simulink model "Model_V9"  (R2024a)
settings: Solver=FixedStepAuto  StartTime=0.0  StopTime=15  FixedStep=10^-3  RelTol=1e-3
values from neighbouring files (symbols this model uses):
  a1 = 1.6552    [varglobal.m]
  a2 = 1.885    [varglobal.m]
  b1 = 0.71    [varglobal.m]
  b2 = 0.71    [varglobal.m]
  Ga1 = 1/7    (= 0.142857142857)    [varglobal.m]
  Gu1 = 1.8    [varglobal.m]
  Gv1 = 1/0.5    (= 2)    [varglobal.m]
  Gx1 = 1/0.5    (= 2)    [varglobal.m]
undefined symbols (not defined in the file or in its folder): eqmovimento, Forcalateral, ForcaMolaFrontal, ForcaMolaRetaguarda, Rotacao, Saidas, sigbuilder_block, Transformador, TransformadorT
libraries: simulink_extras x5, fuzblock x4
settings Model: Creator=Vilson Wenis Belle  LastModifiedBy=wenis
settings SolverCC: AlgebraicLoopSolver=TrustRegion
settings DebuggingCC: UnconnectedInputMsg=warning  UnconnectedOutputMsg=warning  UnconnectedLineMsg=warning
settings ModelReferenceCC: EnableRefExpFcnMdlSchedulingChecks=on
settings RTWCC: GPUComputeCapability=3.5

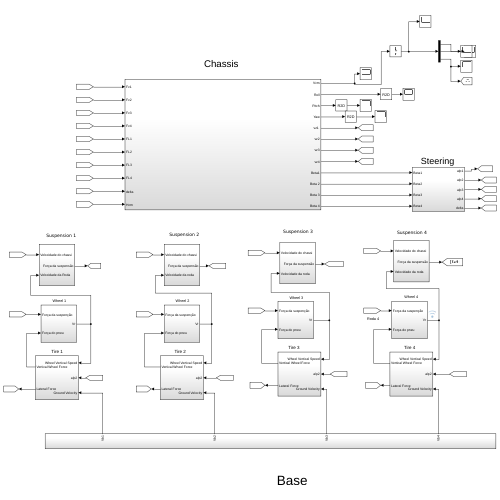
[thumbnail: Simulink's stored preview of the top-level diagram]
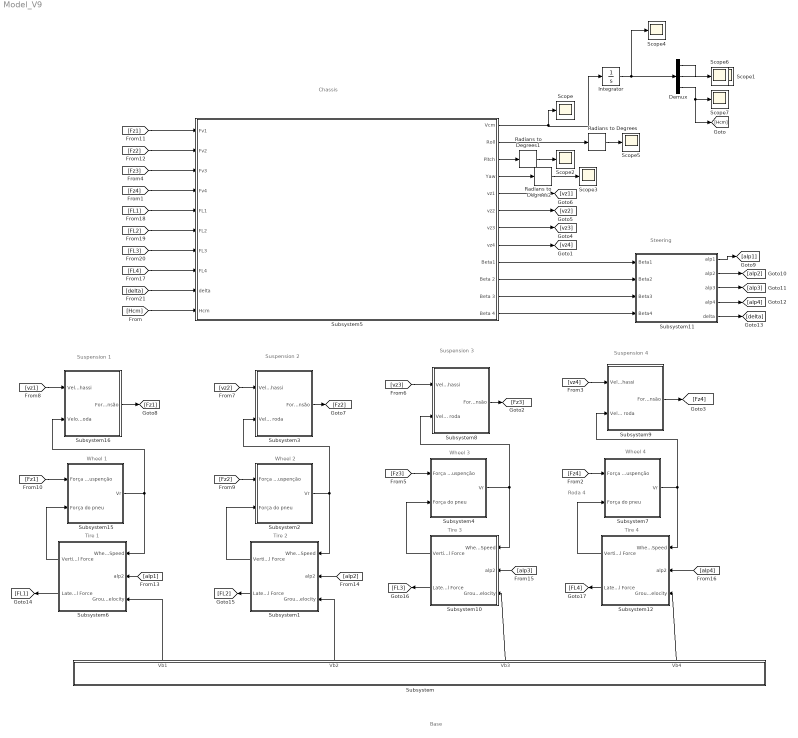
== system Model_V9 ==
  note: Chassis
  note: Steering
  note: Suspension 4
  note: Roda 4
  note: Tire 4
  note: Suspension 3
  note: Wheel 3
  note: Suspension 2
  note: Wheel 2
  note: Base
  note: Suspension 1
  note: Wheel 1
  note: Tire 3
  note: Tire 2
  note: Tire 1
  note: Wheel 4
  Demux : Demux  Outputs=3
  Integrator : Integrator  InitialCondition=[0 (1.1*1.4 + 0.25)/2 0.6]
  Radians to Degrees : simulink_extras/Transformations/Radians to Degrees
  Radians to Degrees1 : simulink_extras/Transformations/Radians to Degrees
  Radians to Degrees2 : simulink_extras/Transformations/Radians to Degrees
  Scope{,1..7} (8 alike) : Scope
  Subsystem : Subsystem
  Subsystem1 : Subsystem
  Subsystem10 : Subsystem
  Subsystem11 : Subsystem
  Subsystem12 : Subsystem
  Subsystem15 : Subsystem
  Subsystem16 : Subsystem
  Subsystem2 : Subsystem
  Subsystem3 : Subsystem
  Subsystem4 : Subsystem
  Subsystem5 : Subsystem
  Subsystem6 : Subsystem
  Subsystem7 : Subsystem
  Subsystem8 : Subsystem
  Subsystem9 : Subsystem
  wires:
  Subsystem12/1(Vertical Wheel Force) -> Subsystem7/2(Força do pneu)
  Subsystem7/1(Vr) -> Subsystem12/1(Wheel Vertical Speed), Subsystem9/2(Velocidade da roda)
  Subsystem4/1(Vr) -> Subsystem10/1(Wheel Vertical Speed), Subsystem8/2(Velocidade da roda)
  Subsystem10/1(Vertical Wheel Force) -> Subsystem4/2(Força do pneu)
  Subsystem2/1(Vr) -> Subsystem1/1(Wheel Vertical Speed), Subsystem3/2(Velocidade da roda)
  Subsystem1/1(Vertical Wheel Force) -> Subsystem2/2(Força do pneu)
  Subsystem15/1(Vr) -> Subsystem6/1(Wheel Vertical Speed), Subsystem16/2(Velocidade da Roda)
  Subsystem9/1(Força da suspensão) -> [Fz4]
  Subsystem5/1(Vcm) -> Scope/1, Integrator/1
  Subsystem5/2(Roll) -> Radians to Degrees/1
  Subsystem5/3(Pitch) -> Radians to Degrees1/1
  Subsystem5/4(Yaw) -> Radians to Degrees2/1
  Integrator/1 -> Scope4/1, Demux/1
  Subsystem6/1(Vertical Wheel Force) -> Subsystem15/2(Força do pneu)
  [Fz4] -> Subsystem5/4(Fv4)
  [Fz4] -> Subsystem7/1(Força da suspenção)
  Subsystem5/8(vz4) -> [vz4]
  [vz4] -> Subsystem9/1(Velocidade do chassi)
  [Fz3] -> Subsystem5/3(Fv3)
  Subsystem8/1(Força da suspensão) -> [Fz3]
  [Fz3] -> Subsystem4/1(Força da suspenção)
  Subsystem5/7(vz3) -> [vz3]
  [vz3] -> Subsystem8/1(Velocidade do chassi)
  Subsystem5/6(vz2) -> [vz2]
  Subsystem5/5("vz1 ") -> [vz1]
  [vz2] -> Subsystem3/1(Velocidade do chassi)
  [vz1] -> Subsystem16/1(Velocidade do chassi)
  Subsystem3/1(Força da suspensão) -> [Fz2]
  Subsystem16/1(Força da suspensão) -> [Fz1]
  [Fz2] -> Subsystem2/1(Força da suspenção)
  [Fz1] -> Subsystem15/1(Força da suspenção)
  [Fz1] -> Subsystem5/1(Fv1)
  [Fz2] -> Subsystem5/2(Fv2)
  Subsystem/1(Vb1) -> Subsystem6/3(Ground Velocity)
  Subsystem/2(Vb2) -> Subsystem1/3(Ground Velocity)
  Subsystem/3(Vb3) -> Subsystem10/3(Ground Velocity)
  Subsystem/4(Vb4) -> Subsystem12/3(Ground Velocity)
  Subsystem5/9(Beta1) -> Subsystem11/1("Beta1 ")
  Subsystem5/10(Beta 2) -> Subsystem11/2(Beta2)
  Subsystem5/11(Beta 3) -> Subsystem11/3(Beta3)
  Subsystem5/12(Beta 4) -> Subsystem11/4(Beta4)
  [alp1] -> Subsystem6/2(alp2)
  Subsystem11/1(alp1) -> [alp1]
  Subsystem11/2(alp2) -> [alp2]
  Subsystem11/3(alp3) -> [alp3]
  Subsystem11/4(alp4) -> [alp4]
  Subsystem11/5(delta) -> [delta]
  [alp2] -> Subsystem1/2(alp2)
  [alp3] -> Subsystem10/2(alp2)
  [alp4] -> Subsystem12/2(alp2)
  Subsystem6/2(Lateral Force) -> [FL1]
  Subsystem1/2(Lateral Force) -> [FL2]
  Subsystem10/2(Lateral Force) -> [FL3]
  Subsystem12/2(Lateral Force) -> [FL4]
  [FL1] -> Subsystem5/5(FL1)
  [FL2] -> Subsystem5/6(FL2)
  [FL3] -> Subsystem5/7(FL3)
  [FL4] -> Subsystem5/8(FL4)
  [delta] -> Subsystem5/9(delta)
  Radians to Degrees1/1 -> Scope2/1
  Demux/1 -> Scope1/1
  Demux/2 -> Scope6/1
  Demux/3 -> [Hcm], Scope7/1
  [Hcm] -> Subsystem5/10("Hcm ")
  Radians to Degrees2/1 -> Scope3/1
  Radians to Degrees/1 -> Scope5/1

== system Model_V9/Subsystem ==
  Signal Builder : Subsystem  Tag=STV Subsys  LoadFcn=sigbuilder_block('load');  StartFcn=sigbuilder_block('start');  StopFcn=sigbuilder_block('stop');  ClipboardFcn=sigbuilder_block('clipboard');  mask(Sigbuilder block){tuvar=[0:10]}
      mask help: Simulink:masks:SigbuilderBlock_MD
      mask init:
      | if ~strcmp(get_param(bdroot(gcbh),'SimulationStatus'),'stopped') tuvar = sigbuilder_block('maskInit'); end
      settings: CopyFcn=sigbuilder_block('copy');  DeleteFcn=sigbuilder_block('delete');  ModelCloseFcn=sigbuilder_block('modelClose');  PreSaveFcn=sigbuilder_block('preSave');  PauseFcn=sigbuilder_block('pause');  ContinueFcn=sigbuilder_block('continue');  NameChangeFcn=sigbuilder_block('namechange');  OpenFcn=sigbuilder_block('open',[437.25 153 550.5 359.25 ]);  CloseFcn=sigbuilder_block('close');
      mask Display: plot(0, 0, 100, 100,[2, 2, 32, 32, 2], [68, 8, 8, 68, 68],[32, 2], [38, 38], [32, 19, 2],[53, 60, 44], [32, 17, 17, 2],[16, 16, 31, 31]);txt = getActiveGroup(gcbh);text(2, 100, txt,'verticalAlignment', 'top');
  Vb1 : Outport
  Vb2 : Outport  Port=2
  Vb3 : Outport  Port=3
  Vb4 : Outport  Port=4
  wires:
  Signal Builder/1(Signal 1) -> Vb1/1
  Signal Builder/2(Signal 2) -> Vb2/1
  Signal Builder/3(Signal 3) -> Vb3/1
  Signal Builder/4(Signal 4) -> Vb4/1

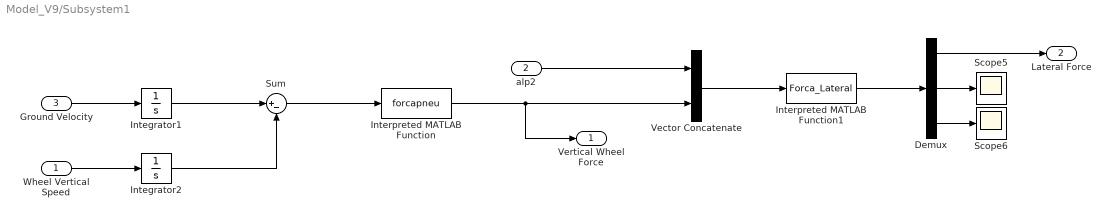
== system Model_V9/Subsystem1 ==
  Wheel Vertical Speed : Inport
  alp2 : Inport  Port=2
  Ground Velocity : Inport  Port=3
  Demux : Demux  Outputs=3
  Integrator1 : Integrator
  Integrator2 : Integrator
  Interpreted MATLAB Function : MATLABFcn  MATLABFcn=forcapneu  OutputDimensions=1
  Interpreted MATLAB Function1 : MATLABFcn  MATLABFcn=Forca_Lateral  OutputDimensions=3
  Scope5 : Scope
  Scope6 : Scope
  Sum : Sum  Inputs=|+-
  Vector Concatenate : Concatenate
  Vertical Wheel Force : Outport
  Lateral Force : Outport  Port=2
  wires:
  Ground Velocity/1 -> Integrator1/1
  Integrator2/1 -> Sum/2
  Interpreted MATLAB Function/1 -> Vertical Wheel Force/1, Vector Concatenate/2
  Integrator1/1 -> Sum/1
  Wheel Vertical Speed/1 -> Integrator2/1
  Sum/1 -> Interpreted MATLAB Function/1
  alp2/1 -> Vector Concatenate/1
  Vector Concatenate/1 -> Interpreted MATLAB Function1/1
  Interpreted MATLAB Function1/1 -> Demux/1
  Demux/1 -> Lateral Force/1
  Demux/2 -> Scope5/1
  Demux/3 -> Scope6/1

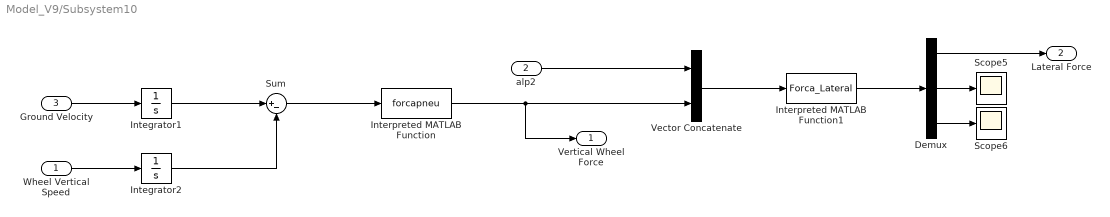
== system Model_V9/Subsystem10 ==
  Wheel Vertical Speed : Inport
  alp2 : Inport  Port=2
  Ground Velocity : Inport  Port=3
  Demux : Demux  Outputs=3
  Integrator1 : Integrator
  Integrator2 : Integrator
  Interpreted MATLAB Function : MATLABFcn  MATLABFcn=forcapneu  OutputDimensions=1
  Interpreted MATLAB Function1 : MATLABFcn  MATLABFcn=Forca_Lateral  OutputDimensions=3
  Scope5 : Scope
  Scope6 : Scope
  Sum : Sum  Inputs=|+-
  Vector Concatenate : Concatenate
  Vertical Wheel Force : Outport
  Lateral Force : Outport  Port=2
  wires:
  Ground Velocity/1 -> Integrator1/1
  Integrator2/1 -> Sum/2
  Interpreted MATLAB Function/1 -> Vertical Wheel Force/1, Vector Concatenate/2
  Integrator1/1 -> Sum/1
  Wheel Vertical Speed/1 -> Integrator2/1
  Sum/1 -> Interpreted MATLAB Function/1
  alp2/1 -> Vector Concatenate/1
  Vector Concatenate/1 -> Interpreted MATLAB Function1/1
  Interpreted MATLAB Function1/1 -> Demux/1
  Demux/1 -> Lateral Force/1
  Demux/2 -> Scope5/1
  Demux/3 -> Scope6/1

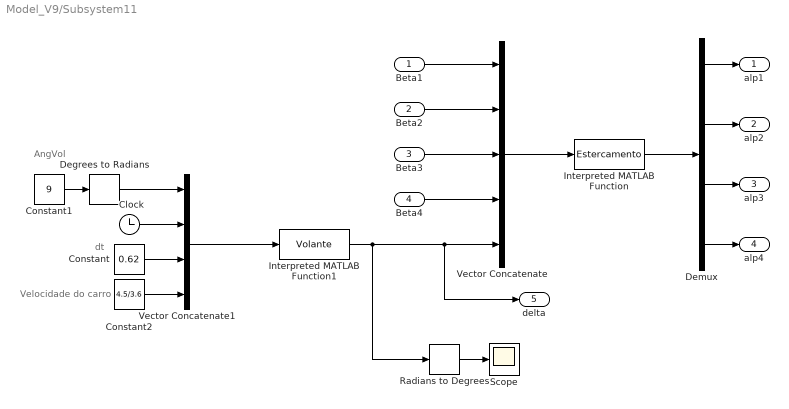
== system Model_V9/Subsystem11 ==
  note: Velocidade do carro
  note: dt
  note: AngVol
  "Beta1 " : Inport
  Beta2 : Inport  Port=2
  Beta3 : Inport  Port=3
  Beta4 : Inport  Port=4
  Clock : Clock
  Constant : Constant  Value=0.62
  Constant1 : Constant  Value=9
  Constant2 : Constant  Value=4.5/3.6
  Degrees to Radians : simulink_extras/Transformations/Degrees to Radians
  Demux : Demux
  Interpreted MATLAB Function : MATLABFcn  MATLABFcn=Estercamento  OutputDimensions=4
  Interpreted MATLAB Function1 : MATLABFcn  MATLABFcn=Volante  OutputDimensions=1
  Radians to Degrees : simulink_extras/Transformations/Radians to Degrees
  Scope : Scope
  Vector Concatenate : Concatenate  NumInputs=5
  Vector Concatenate1 : Concatenate  NumInputs=4
  alp1 : Outport
  alp2 : Outport  Port=2
  alp3 : Outport  Port=3
  alp4 : Outport  Port=4
  delta : Outport  Port=5
  wires:
  Beta4/1 -> Vector Concatenate/4
  Beta3/1 -> Vector Concatenate/3
  Beta2/1 -> Vector Concatenate/2
  "Beta1 "/1 -> Vector Concatenate/1
  Vector Concatenate/1 -> Interpreted MATLAB Function/1
  Interpreted MATLAB Function/1 -> Demux/1
  Demux/1 -> alp1/1
  Demux/2 -> alp2/1
  Demux/3 -> alp3/1
  Demux/4 -> alp4/1
  Clock/1 -> Vector Concatenate1/2
  Constant1/1 -> Degrees to Radians/1
  Constant/1 -> Vector Concatenate1/3
  Vector Concatenate1/1 -> Interpreted MATLAB Function1/1
  Degrees to Radians/1 -> Vector Concatenate1/1
  Constant2/1 -> Vector Concatenate1/4
  Radians to Degrees/1 -> Scope/1
  Interpreted MATLAB Function1/1 -> delta/1, Vector Concatenate/5, Radians to Degrees/1

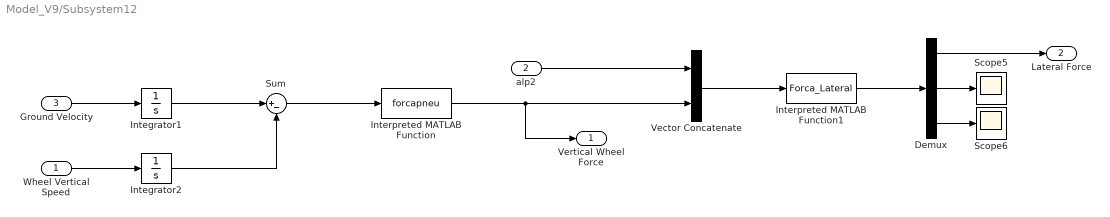
== system Model_V9/Subsystem12 ==
  Wheel Vertical Speed : Inport
  alp2 : Inport  Port=2
  Ground Velocity : Inport  Port=3
  Demux : Demux  Outputs=3
  Integrator1 : Integrator
  Integrator2 : Integrator
  Interpreted MATLAB Function : MATLABFcn  MATLABFcn=forcapneu  OutputDimensions=1
  Interpreted MATLAB Function1 : MATLABFcn  MATLABFcn=Forca_Lateral  OutputDimensions=3
  Scope5 : Scope
  Scope6 : Scope
  Sum : Sum  Inputs=|+-
  Vector Concatenate : Concatenate
  Vertical Wheel Force : Outport
  Lateral Force : Outport  Port=2
  wires:
  Ground Velocity/1 -> Integrator1/1
  Integrator2/1 -> Sum/2
  Interpreted MATLAB Function/1 -> Vertical Wheel Force/1, Vector Concatenate/2
  Integrator1/1 -> Sum/1
  Wheel Vertical Speed/1 -> Integrator2/1
  Sum/1 -> Interpreted MATLAB Function/1
  alp2/1 -> Vector Concatenate/1
  Vector Concatenate/1 -> Interpreted MATLAB Function1/1
  Interpreted MATLAB Function1/1 -> Demux/1
  Demux/1 -> Lateral Force/1
  Demux/2 -> Scope5/1
  Demux/3 -> Scope6/1

== system Model_V9/Subsystem15 ==
  Força da suspenção : Inport
  Força do pneu : Inport  Port=2
  Integrator : Integrator
  Interpreted MATLAB Function1 : MATLABFcn  MATLABFcn=aceleracaorodafrontal  OutputDimensions=1
  Sum : Sum  Inputs=|-+
  Vr : Outport
  wires:
  Força da suspenção/1 -> Sum/1
  Força do pneu/1 -> Sum/2
  Integrator/1 -> Vr/1
  Sum/1 -> Interpreted MATLAB Function1/1
  Interpreted MATLAB Function1/1 -> Integrator/1

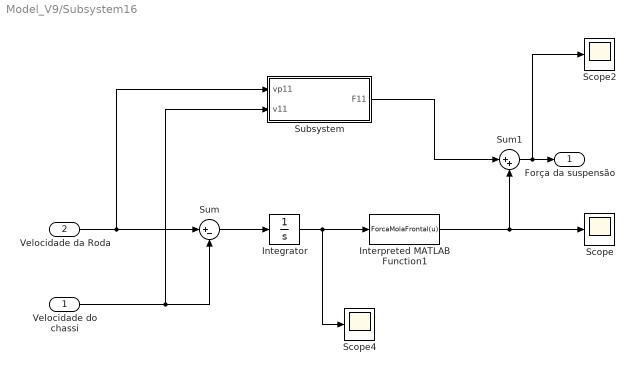
== system Model_V9/Subsystem16 ==
  Velocidade do chassi : Inport
  Velocidade da Roda : Inport  Port=2
  Integrator : Integrator
  Interpreted MATLAB Function1 : MATLABFcn  MATLABFcn=ForcaMolaFrontal(u)  OutputDimensions=1
  Scope : Scope
  Scope2 : Scope
  Scope4 : Scope
  Subsystem : Subsystem
  Sum : Sum  Inputs=|+-
  Sum1 : Sum  Inputs=|++
  Força da suspensão : Outport
  wires:
  Velocidade do chassi/1 -> Subsystem/2(v11), Sum/2
  Velocidade da Roda/1 -> Subsystem/1(vp11), Sum/1
  Sum/1 -> Integrator/1
  Integrator/1 -> Scope4/1, Interpreted MATLAB Function1/1
  Interpreted MATLAB Function1/1 -> Scope/1, Sum1/2
  Sum1/1 -> Scope2/1, Força da suspensão/1
  Subsystem/1(F11) -> Sum1/1

== system Model_V9/Subsystem2 ==
  Força da suspenção : Inport
  Força do pneu : Inport  Port=2
  Integrator : Integrator
  Interpreted MATLAB Function : MATLABFcn  MATLABFcn=aceleracaorodafrontal  OutputDimensions=1
  Sum : Sum  Inputs=|-+
  Vr : Outport
  wires:
  Força da suspenção/1 -> Sum/1
  Força do pneu/1 -> Sum/2
  Integrator/1 -> Vr/1
  Sum/1 -> Interpreted MATLAB Function/1
  Interpreted MATLAB Function/1 -> Integrator/1

== system Model_V9/Subsystem3 ==
  Velocidade do chassi : Inport
  Velocidade da roda : Inport  Port=2
  Integrator : Integrator
  Interpreted MATLAB Function1 : MATLABFcn  MATLABFcn=ForcaMolaFrontal(u)  OutputDimensions=1
  Scope : Scope
  Scope1 : Scope
  Scope2 : Scope
  Subsystem : Subsystem
  Sum : Sum  Inputs=|+-
  Sum1 : Sum  Inputs=|++
  Força da suspensão : Outport
  wires:
  Velocidade do chassi/1 -> Subsystem/2(v11), Sum/2
  Velocidade da roda/1 -> Sum/1, Subsystem/1(vp11)
  Sum/1 -> Integrator/1
  Integrator/1 -> Interpreted MATLAB Function1/1, Scope/1
  Sum1/1 -> Scope1/1, Força da suspensão/1
  Interpreted MATLAB Function1/1 -> Scope2/1, Sum1/2
  Subsystem/1(F11) -> Sum1/1

== system Model_V9/Subsystem4 ==
  Força da suspenção : Inport
  Força do pneu : Inport  Port=2
  Integrator : Integrator
  Interpreted MATLAB Function : MATLABFcn  MATLABFcn=aceleracaorodaretaguarda  OutputDimensions=1
  Sum : Sum  Inputs=|-+
  Vr : Outport
  wires:
  Força da suspenção/1 -> Sum/1
  Força do pneu/1 -> Sum/2
  Integrator/1 -> Vr/1
  Sum/1 -> Interpreted MATLAB Function/1
  Interpreted MATLAB Function/1 -> Integrator/1

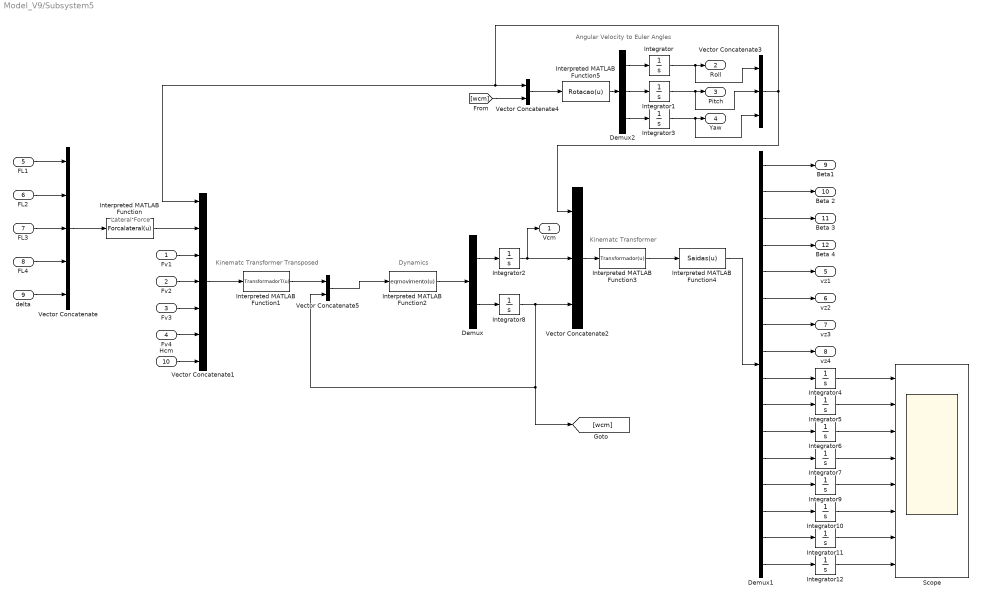
== system Model_V9/Subsystem5 ==
  note: Angular Velocity to Euler Angles
  note: Kinematc Transformer Transposed
  note: Dynamics
  note: Lateral Force
  note: Kinematc Transformer
  Fv1 : Inport
  Fv2 : Inport  Port=2
  Fv3 : Inport  Port=3
  Fv4 : Inport  Port=4
  FL1 : Inport  Port=5
  FL2 : Inport  Port=6
  FL3 : Inport  Port=7
  FL4 : Inport  Port=8
  delta : Inport  Port=9
  "Hcm " : Inport  Port=10
  Demux : Demux  Outputs=2
  Demux1 : Demux  Outputs=16
  Demux2 : Demux  Outputs=3
  Integrator : Integrator
  Integrator1 : Integrator
  Integrator10 : Integrator  InitialCondition=(1.1*1.4 + 0.25)/2+b1
  Integrator11 : Integrator  InitialCondition=-a2
  Integrator12 : Integrator  InitialCondition=(1.1*1.4 + 0.25)/2-b2
  Integrator2 : Integrator  InitialCondition=[60/3.6 0 0]
  Integrator3 : Integrator
  Integrator4 : Integrator  InitialCondition=a1
  Integrator5 : Integrator  InitialCondition=(1.1*1.4 + 0.25)/2+b1
  Integrator6 : Integrator  InitialCondition=a1
  Integrator7 : Integrator  InitialCondition=(1.1*1.4 + 0.25)/2-b2
  Integrator8 : Integrator  InitialCondition=[0 0 0]
  Integrator9 : Integrator  InitialCondition=-a2
  Interpreted MATLAB Function : MATLABFcn  MATLABFcn=Forcalateral(u)  OutputDimensions=6
  Interpreted MATLAB Function1 : MATLABFcn  MATLABFcn=TransformadorT(u)  OutputDimensions=6
  Interpreted MATLAB Function2 : MATLABFcn  MATLABFcn=eqmovimento(u)  OutputDimensions=6
  Interpreted MATLAB Function3 : MATLABFcn  MATLABFcn=Transformador(u)  OutputDimensions=13
  Interpreted MATLAB Function4 : MATLABFcn  MATLABFcn=Saidas(u)  OutputDimensions=16
  Interpreted MATLAB Function5 : MATLABFcn  MATLABFcn=Rotacao(u)  OutputDimensions=3
  Scope : Scope  NumInputPorts=8
  Vector Concatenate : Concatenate  NumInputs=5
  Vector Concatenate1 : Concatenate  NumInputs=7
  Vector Concatenate2 : Concatenate  NumInputs=3
  Vector Concatenate3 : Concatenate  NumInputs=3
  Vector Concatenate4 : Concatenate
  Vector Concatenate5 : Concatenate
  Vcm : Outport
  Roll : Outport  Port=2
  Pitch : Outport  Port=3
  Yaw : Outport  Port=4
  "vz1 " : Outport  Port=5
  vz2 : Outport  Port=6
  vz3 : Outport  Port=7
  vz4 : Outport  Port=8
  Beta1 : Outport  Port=9
  Beta 2 : Outport  Port=10
  Beta 3 : Outport  Port=11
  Beta 4 : Outport  Port=12
  wires:
  Demux1/1 -> Beta1/1
  Demux1/2 -> Beta 2/1
  Demux1/3 -> Beta 3/1
  Demux1/4 -> Beta 4/1
  Demux1/6 -> vz2/1
  Demux1/5 -> "vz1 "/1
  Demux1/7 -> vz3/1
  Demux1/8 -> vz4/1
  Vector Concatenate/1 -> Interpreted MATLAB Function/1
  Vector Concatenate1/1 -> Interpreted MATLAB Function1/1
  Fv4/1 -> Vector Concatenate1/6
  Fv3/1 -> Vector Concatenate1/5
  Interpreted MATLAB Function2/1 -> Demux/1
  Demux/1 -> Integrator2/1
  Demux/2 -> Integrator8/1
  Vector Concatenate2/1 -> Interpreted MATLAB Function3/1
  Interpreted MATLAB Function3/1 -> Interpreted MATLAB Function4/1
  Interpreted MATLAB Function4/1 -> Demux1/1
  Interpreted MATLAB Function5/1 -> Demux2/1
  Demux2/1 -> Integrator/1
  Demux2/2 -> Integrator1/1
  Demux2/3 -> Integrator3/1
  Integrator/1 -> Vector Concatenate3/1, Roll/1
  Integrator1/1 -> Vector Concatenate3/2, Pitch/1
  Integrator3/1 -> Vector Concatenate3/3, Yaw/1
  Interpreted MATLAB Function/1 -> Vector Concatenate1/2
  Fv1/1 -> Vector Concatenate1/3
  Fv2/1 -> Vector Concatenate1/4
  Integrator2/1 -> Vcm/1, Vector Concatenate2/2
  Vector Concatenate3/1 -> Vector Concatenate2/1, Vector Concatenate4/1, Vector Concatenate1/1
  Vector Concatenate4/1 -> Interpreted MATLAB Function5/1
  FL1/1 -> Vector Concatenate/1
  FL2/1 -> Vector Concatenate/2
  FL3/1 -> Vector Concatenate/3
  FL4/1 -> Vector Concatenate/4
  delta/1 -> Vector Concatenate/5
  "Hcm "/1 -> Vector Concatenate1/7
  [wcm] -> Vector Concatenate4/2
  Demux1/9 -> Integrator4/1
  Demux1/10 -> Integrator5/1
  Demux1/11 -> Integrator6/1
  Demux1/12 -> Integrator7/1
  Demux1/13 -> Integrator9/1
  Demux1/14 -> Integrator10/1
  Demux1/15 -> Integrator11/1
  Demux1/16 -> Integrator12/1
  Integrator4/1 -> Scope/1
  Integrator5/1 -> Scope/2
  Integrator6/1 -> Scope/3
  Integrator7/1 -> Scope/4
  Integrator9/1 -> Scope/5
  Integrator10/1 -> Scope/6
  Integrator11/1 -> Scope/7
  Integrator12/1 -> Scope/8
  Integrator8/1 -> Vector Concatenate5/2, [wcm], Vector Concatenate2/3
  Interpreted MATLAB Function1/1 -> Vector Concatenate5/1
  Vector Concatenate5/1 -> Interpreted MATLAB Function2/1

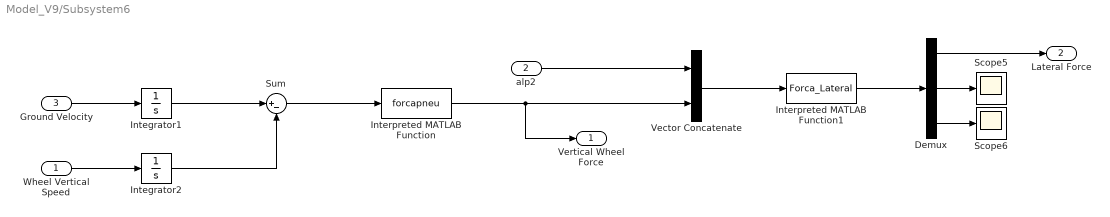
== system Model_V9/Subsystem6 ==
  Wheel Vertical Speed : Inport
  alp2 : Inport  Port=2
  Ground Velocity : Inport  Port=3
  Demux : Demux  Outputs=3
  Integrator1 : Integrator
  Integrator2 : Integrator
  Interpreted MATLAB Function : MATLABFcn  MATLABFcn=forcapneu  OutputDimensions=1
  Interpreted MATLAB Function1 : MATLABFcn  MATLABFcn=Forca_Lateral  OutputDimensions=3
  Scope5 : Scope
  Scope6 : Scope
  Sum : Sum  Inputs=|+-
  Vector Concatenate : Concatenate
  Vertical Wheel Force : Outport
  Lateral Force : Outport  Port=2
  wires:
  Ground Velocity/1 -> Integrator1/1
  Integrator2/1 -> Sum/2
  Interpreted MATLAB Function/1 -> Vertical Wheel Force/1, Vector Concatenate/2
  Integrator1/1 -> Sum/1
  Wheel Vertical Speed/1 -> Integrator2/1
  Sum/1 -> Interpreted MATLAB Function/1
  alp2/1 -> Vector Concatenate/1
  Vector Concatenate/1 -> Interpreted MATLAB Function1/1
  Interpreted MATLAB Function1/1 -> Demux/1
  Demux/1 -> Lateral Force/1
  Demux/2 -> Scope5/1
  Demux/3 -> Scope6/1

== system Model_V9/Subsystem7 ==
  Força da suspenção : Inport
  Força do pneu : Inport  Port=2
  Integrator : Integrator
  Interpreted MATLAB Function : MATLABFcn  MATLABFcn=aceleracaorodaretaguarda  OutputDimensions=1
  Sum : Sum  Inputs=|-+
  Vr : Outport
  wires:
  Força da suspenção/1 -> Sum/1
  Força do pneu/1 -> Sum/2
  Integrator/1 -> Vr/1
  Sum/1 -> Interpreted MATLAB Function/1
  Interpreted MATLAB Function/1 -> Integrator/1

== system Model_V9/Subsystem8 ==
  Velocidade do chassi : Inport
  Velocidade da roda : Inport  Port=2
  Integrator : Integrator
  Interpreted MATLAB Function1 : MATLABFcn  MATLABFcn=ForcaMolaRetaguarda(u)  OutputDimensions=1
  Scope1 : Scope
  Scope2 : Scope
  Scope3 : Scope
  Subsystem : Subsystem
  Sum : Sum  Inputs=|+-
  Sum1 : Sum  Inputs=|++
  Força da suspensão : Outport
  wires:
  Velocidade do chassi/1 -> Subsystem/2(v11), Sum/2
  Velocidade da roda/1 -> Subsystem/1(vp11), Sum/1
  Sum/1 -> Integrator/1
  Subsystem/1(F11) -> Sum1/1
  Interpreted MATLAB Function1/1 -> Scope3/1, Sum1/2
  Sum1/1 -> Scope2/1, Força da suspensão/1
  Integrator/1 -> Scope1/1, Interpreted MATLAB Function1/1

== system Model_V9/Subsystem9 ==
  Velocidade do chassi : Inport
  Velocidade da roda : Inport  Port=2
  Integrator : Integrator
  Interpreted MATLAB Function1 : MATLABFcn  MATLABFcn=ForcaMolaRetaguarda(u)  OutputDimensions=1
  Scope1 : Scope
  Scope2 : Scope
  Scope3 : Scope
  Subsystem : Subsystem
  Sum : Sum  Inputs=|+-
  Sum1 : Sum  Inputs=|++
  Força da suspensão : Outport
  wires:
  Velocidade do chassi/1 -> Subsystem/2(v11), Sum/2
  Velocidade da roda/1 -> Sum/1, Subsystem/1(vp11)
  Sum/1 -> Integrator/1
  Sum1/1 -> Scope2/1, Força da suspensão/1
  Integrator/1 -> Scope1/1, Interpreted MATLAB Function1/1
  Interpreted MATLAB Function1/1 -> Scope3/1, Sum1/2
  Subsystem/1(F11) -> Sum1/1

== system Model_V9/Subsystem/Signal Builder ==
  Demux : Demux  Tag=STV Demux
      settings: DisplayOption=none
  FromWs : FromWorkspace  Tag=STV FromWs  VariableName=tuvar
      SigBuilderData=|
      | common.afterFinalStr = 'Extrapolate'
      | common.sampleTime = 0
      | dataSet.timeRange = [0 10]
      | dataSet.name = 'Group 1'
      | sbobj.Groups.Name = 'Group 1'
      | sbobj.Groups.Signals(1).Name = 'Signal 1'
      | sbobj.Groups.Signals(1).XData = [0 4 6 10]
      | sbobj.Groups.Signals(1).YData = [0 0 0 0]
      | sbobj.Groups.Signals(2).Name = 'Signal 2'
      | sbobj.Groups.Signals(2).XData = [0 10]
      | sbobj.Groups.Signals(2).YData = [0 0]
      | sbobj.Groups.Signals(3).Name = 'Signal 3'
      | sbobj.Groups.Signals(3).XData = [0 10]
      | sbobj.Groups.Signals(3).YData = [0 0]
      | sbobj.Groups.Signals(4).Name = 'Signal 4'
      | sbobj.Groups.Signals(4).XData = [0 10]
      | sbobj.Groups.Signals(4).YData = [0 0]
  Signal 1 : Outport  Tag=STV Outport
  Signal 2 : Outport  Tag=STV Outport  Port=2
  Signal 3 : Outport  Tag=STV Outport  Port=3
  Signal 4 : Outport  Tag=STV Outport  Port=4
  wires:
  Demux/1 -> Signal 1/1
  FromWs/1 -> Demux/1
  Demux/2 -> Signal 2/1
  Demux/3 -> Signal 3/1
  Demux/4 -> Signal 4/1

== system Model_V9/Subsystem16/Subsystem ==
  vp11 : Inport
  v11 : Inport  Port=2
  Fuzzy Controller : Subsystem
  "Mag Damper " : Subsystem
  Scope : Scope
  Scope1 : Scope
  To Workspace : ToWorkspace  VariableName=Corrente11  SaveFormat=Timeseries  SampleTime=-1
  F11 : Outport  VectorParamsAs1DForOutWhenUnconnected=off
  wires:
  "Mag Damper "/1(Fb) -> Scope1/1, F11/1
  vp11/1 -> "Mag Damper "/1("Zp_pt "), Fuzzy Controller/2(vp11)
  Fuzzy Controller/1(I1) -> Scope/1, To Workspace/1, "Mag Damper "/3(I)
  v11/1 -> "Mag Damper "/2("Zc_pt "), Fuzzy Controller/1(v11)

== system Model_V9/Subsystem3/Subsystem ==
  vp11 : Inport
  v11 : Inport  Port=2
  "Amortecedor Magnetorreológico " : Subsystem
  Controle Nebuloso : Subsystem
  Scope : Scope
  Scope1 : Scope
  F11 : Outport  VectorParamsAs1DForOutWhenUnconnected=off
  wires:
  "Amortecedor Magnetorreológico "/1(Fb) -> Scope1/1, F11/1
  vp11/1 -> "Amortecedor Magnetorreológico "/1("Zp_pt "), Controle Nebuloso/2(vp11)
  Controle Nebuloso/1(I1) -> Scope/1, "Amortecedor Magnetorreológico "/3(I)
  v11/1 -> "Amortecedor Magnetorreológico "/2("Zc_pt "), Controle Nebuloso/1(v11)

== system Model_V9/Subsystem8/Subsystem ==
  vp11 : Inport
  v11 : Inport  Port=2
  "Amortecedor Magnetorreológico " : Subsystem
  Controle Nebuloso : Subsystem
  Scope : Scope
  Scope1 : Scope
  F11 : Outport  VectorParamsAs1DForOutWhenUnconnected=off
  wires:
  "Amortecedor Magnetorreológico "/1(Fb) -> Scope1/1, F11/1
  vp11/1 -> "Amortecedor Magnetorreológico "/1("Zp_pt "), Controle Nebuloso/2(vp11)
  Controle Nebuloso/1(I1) -> Scope/1, "Amortecedor Magnetorreológico "/3(I)
  v11/1 -> "Amortecedor Magnetorreológico "/2("Zc_pt "), Controle Nebuloso/1(v11)

== system Model_V9/Subsystem9/Subsystem ==
  vp11 : Inport
  v11 : Inport  Port=2
  "Amortecedor Magnetorreológico " : Subsystem
  Controle Nebuloso : Subsystem
  Scope : Scope
  Scope1 : Scope
  F11 : Outport  VectorParamsAs1DForOutWhenUnconnected=off
  wires:
  "Amortecedor Magnetorreológico "/1(Fb) -> Scope1/1, F11/1
  vp11/1 -> "Amortecedor Magnetorreológico "/1("Zp_pt "), Controle Nebuloso/2(vp11)
  Controle Nebuloso/1(I1) -> Scope/1, "Amortecedor Magnetorreológico "/3(I)
  v11/1 -> "Amortecedor Magnetorreológico "/2("Zc_pt "), Controle Nebuloso/1(v11)

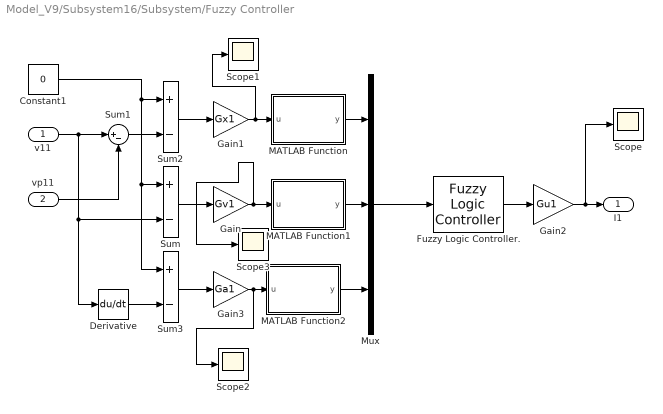
== system Model_V9/Subsystem16/Subsystem/Fuzzy Controller ==
  v11 : Inport
  vp11 : Inport  Port=2
  Constant1 : Constant  Value=0
  Derivative : Derivative
  Fuzzy Logic Controller. : fuzblock/Fuzzy Logic  Controller  FIS='Fuzzy_Sugeno.fis'  OutputSampleNumber=101  DataType=double  FuzzifiedInputs=off  RuleFiringStrengths=off  RuleOutputs=off  AggregatedOutputs=off  SimulateUsing=Interpreted execution  OutOfRangeInputValueMessage=warning  NoRuleFiredMessage=warning  EmptyOutputFuzzySetMessage=warning
  Gain : Gain  Gain=Gv1
  Gain1 : Gain  Gain=Gx1
  Gain2 : Gain  Gain=Gu1
  Gain3 : Gain  Gain=Ga1
  MATLAB Function : MATLAB Function  TreatAsAtomicUnit=on
  MATLAB Function1 : MATLAB Function  TreatAsAtomicUnit=on
  MATLAB Function2 : MATLAB Function  TreatAsAtomicUnit=on
  Mux : Mux  Inputs=3
  Scope{,1..3} (4 alike) : Scope
  Sum : Sum  Inputs=+-
  Sum1 : Sum  Inputs=|+-
  Sum2 : Sum  Inputs=+-
  Sum3 : Sum  Inputs=+-
  I1 : Outport  VectorParamsAs1DForOutWhenUnconnected=off
  wires:
  Constant1/1 -> Sum3/1, Sum/1, Sum2/1
  Sum/1 -> Gain/1
  Sum2/1 -> Gain1/1
  Gain1/1 -> Scope1/1, MATLAB Function/1(u)
  Gain/1 -> MATLAB Function1/1(u), Scope3/1
  v11/1 -> Derivative/1, Sum/2, Sum1/1
  Gain3/1 -> MATLAB Function2/1(u), Scope2/1
  Sum3/1 -> Gain3/1
  Derivative/1 -> Sum3/2
  Gain2/1 -> Scope/1, I1/1
  Fuzzy Logic Controller./1 -> Gain2/1
  Mux/1 -> Fuzzy Logic Controller./1
  vp11/1 -> Sum1/2
  Sum1/1 -> Sum2/2
  MATLAB Function/1(y) -> Mux/1
  MATLAB Function1/1(y) -> Mux/2
  MATLAB Function2/1(y) -> Mux/3

== system Model_V9/Subsystem16/Subsystem/Mag Damper  ==
  "Zp_pt " : Inport
  "Zc_pt " : Inport  Port=2
  I : Inport  Port=3
  Integrator : Integrator
  MR tgh : MATLAB Function  TreatAsAtomicUnit=on
  Sum2 : Sum  Inputs=+-
  Fb : Outport  VectorParamsAs1DForOutWhenUnconnected=off
  wires:
  MR tgh/1(Fb) -> Fb/1
  Integrator/1 -> MR tgh/2(x)
  "Zp_pt "/1 -> Sum2/1
  "Zc_pt "/1 -> Sum2/2
  I/1 -> MR tgh/3(i)
  Sum2/1 -> Integrator/1, MR tgh/1(v)

== system Model_V9/Subsystem3/Subsystem/Amortecedor Magnetorreológico  ==
  "Zp_pt " : Inport
  "Zc_pt " : Inport  Port=2
  I : Inport  Port=3
  Integrator : Integrator
  MR tgh : MATLAB Function  TreatAsAtomicUnit=on
  Sum2 : Sum  Inputs=+-
  Fb : Outport  VectorParamsAs1DForOutWhenUnconnected=off
  wires:
  MR tgh/1(Fb) -> Fb/1
  Integrator/1 -> MR tgh/2(x)
  "Zp_pt "/1 -> Sum2/1
  "Zc_pt "/1 -> Sum2/2
  I/1 -> MR tgh/3(i)
  Sum2/1 -> Integrator/1, MR tgh/1(v)

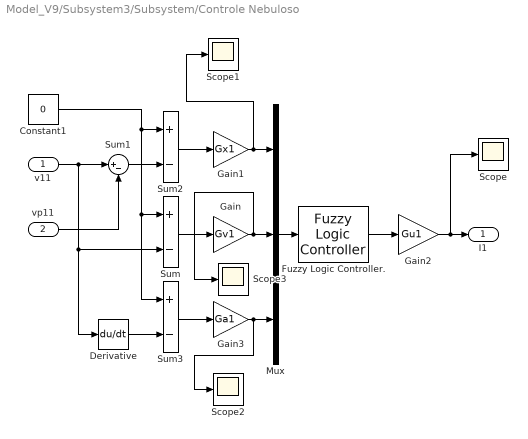
== system Model_V9/Subsystem3/Subsystem/Controle Nebuloso ==
  v11 : Inport
  vp11 : Inport  Port=2
  Constant1 : Constant  Value=0
  Derivative : Derivative
  Fuzzy Logic Controller. : fuzblock/Fuzzy Logic  Controller  FIS='Fuzzy_Sugeno.fis'  OutputSampleNumber=101  DataType=double  FuzzifiedInputs=off  RuleFiringStrengths=off  RuleOutputs=off  AggregatedOutputs=off  SimulateUsing=Interpreted execution  OutOfRangeInputValueMessage=warning  NoRuleFiredMessage=warning  EmptyOutputFuzzySetMessage=warning
  Gain : Gain  Gain=Gv1
  Gain1 : Gain  Gain=Gx1
  Gain2 : Gain  Gain=Gu1
  Gain3 : Gain  Gain=Ga1
  Mux : Mux  Inputs=3
  Scope{,1..3} (4 alike) : Scope
  Sum : Sum  Inputs=+-
  Sum1 : Sum  Inputs=|+-
  Sum2 : Sum  Inputs=+-
  Sum3 : Sum  Inputs=+-
  I1 : Outport  VectorParamsAs1DForOutWhenUnconnected=off
  wires:
  Constant1/1 -> Sum3/1, Sum/1, Sum2/1
  Sum/1 -> Gain/1
  Sum2/1 -> Gain1/1
  Gain1/1 -> Scope1/1, Mux/1
  Gain/1 -> Scope3/1, Mux/2
  v11/1 -> Derivative/1, Sum/2, Sum1/1
  Gain3/1 -> Scope2/1, Mux/3
  Sum3/1 -> Gain3/1
  Derivative/1 -> Sum3/2
  Gain2/1 -> Scope/1, I1/1
  Fuzzy Logic Controller./1 -> Gain2/1
  Mux/1 -> Fuzzy Logic Controller./1
  vp11/1 -> Sum1/2
  Sum1/1 -> Sum2/2

== system Model_V9/Subsystem8/Subsystem/Amortecedor Magnetorreológico  ==
  "Zp_pt " : Inport
  "Zc_pt " : Inport  Port=2
  I : Inport  Port=3
  Integrator : Integrator
  MR tgh : MATLAB Function  TreatAsAtomicUnit=on
  Sum2 : Sum  Inputs=+-
  Fb : Outport  VectorParamsAs1DForOutWhenUnconnected=off
  wires:
  MR tgh/1(Fb) -> Fb/1
  Integrator/1 -> MR tgh/2(x)
  "Zp_pt "/1 -> Sum2/1
  "Zc_pt "/1 -> Sum2/2
  I/1 -> MR tgh/3(i)
  Sum2/1 -> Integrator/1, MR tgh/1(v)

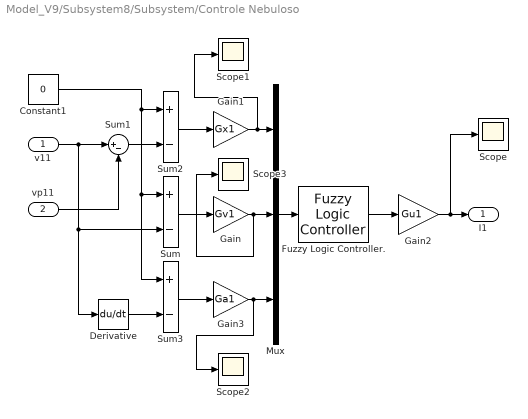
== system Model_V9/Subsystem8/Subsystem/Controle Nebuloso ==
  v11 : Inport
  vp11 : Inport  Port=2
  Constant1 : Constant  Value=0
  Derivative : Derivative
  Fuzzy Logic Controller. : fuzblock/Fuzzy Logic  Controller  FIS='Fuzzy_Sugeno.fis'  OutputSampleNumber=101  DataType=double  FuzzifiedInputs=off  RuleFiringStrengths=off  RuleOutputs=off  AggregatedOutputs=off  SimulateUsing=Interpreted execution  OutOfRangeInputValueMessage=warning  NoRuleFiredMessage=warning  EmptyOutputFuzzySetMessage=warning
  Gain : Gain  Gain=Gv1
  Gain1 : Gain  Gain=Gx1
  Gain2 : Gain  Gain=Gu1
  Gain3 : Gain  Gain=Ga1
  Mux : Mux  Inputs=3
  Scope{,1..3} (4 alike) : Scope
  Sum : Sum  Inputs=+-
  Sum1 : Sum  Inputs=|+-
  Sum2 : Sum  Inputs=+-
  Sum3 : Sum  Inputs=+-
  I1 : Outport  VectorParamsAs1DForOutWhenUnconnected=off
  wires:
  Constant1/1 -> Sum3/1, Sum/1, Sum2/1
  Sum/1 -> Gain/1
  Sum2/1 -> Gain1/1
  Gain1/1 -> Scope1/1, Mux/1
  Gain/1 -> Scope3/1, Mux/2
  v11/1 -> Derivative/1, Sum/2, Sum1/1
  Gain3/1 -> Scope2/1, Mux/3
  Sum3/1 -> Gain3/1
  Derivative/1 -> Sum3/2
  Gain2/1 -> Scope/1, I1/1
  Fuzzy Logic Controller./1 -> Gain2/1
  Mux/1 -> Fuzzy Logic Controller./1
  vp11/1 -> Sum1/2
  Sum1/1 -> Sum2/2

== system Model_V9/Subsystem9/Subsystem/Amortecedor Magnetorreológico  ==
  "Zp_pt " : Inport
  "Zc_pt " : Inport  Port=2
  I : Inport  Port=3
  Integrator : Integrator
  MR tgh : MATLAB Function  TreatAsAtomicUnit=on
  Sum2 : Sum  Inputs=+-
  Fb : Outport  VectorParamsAs1DForOutWhenUnconnected=off
  wires:
  MR tgh/1(Fb) -> Fb/1
  Integrator/1 -> MR tgh/2(x)
  "Zp_pt "/1 -> Sum2/1
  "Zc_pt "/1 -> Sum2/2
  I/1 -> MR tgh/3(i)
  Sum2/1 -> Integrator/1, MR tgh/1(v)

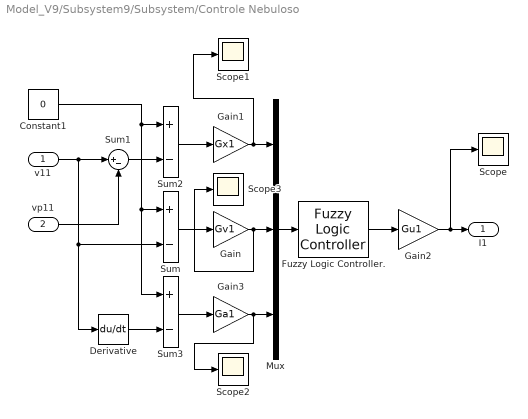
== system Model_V9/Subsystem9/Subsystem/Controle Nebuloso ==
  v11 : Inport
  vp11 : Inport  Port=2
  Constant1 : Constant  Value=0
  Derivative : Derivative
  Fuzzy Logic Controller. : fuzblock/Fuzzy Logic  Controller  FIS='Fuzzy_Sugeno.fis'  OutputSampleNumber=101  DataType=double  FuzzifiedInputs=off  RuleFiringStrengths=off  RuleOutputs=off  AggregatedOutputs=off  SimulateUsing=Interpreted execution  OutOfRangeInputValueMessage=warning  NoRuleFiredMessage=warning  EmptyOutputFuzzySetMessage=warning
  Gain : Gain  Gain=Gv1
  Gain1 : Gain  Gain=Gx1
  Gain2 : Gain  Gain=Gu1
  Gain3 : Gain  Gain=Ga1
  Mux : Mux  Inputs=3
  Scope{,1..3} (4 alike) : Scope
  Sum : Sum  Inputs=+-
  Sum1 : Sum  Inputs=|+-
  Sum2 : Sum  Inputs=+-
  Sum3 : Sum  Inputs=+-
  I1 : Outport  VectorParamsAs1DForOutWhenUnconnected=off
  wires:
  Constant1/1 -> Sum3/1, Sum/1, Sum2/1
  Sum/1 -> Gain/1
  Sum2/1 -> Gain1/1
  Gain1/1 -> Scope1/1, Mux/1
  Gain/1 -> Scope3/1, Mux/2
  v11/1 -> Derivative/1, Sum/2, Sum1/1
  Gain3/1 -> Scope2/1, Mux/3
  Sum3/1 -> Gain3/1
  Derivative/1 -> Sum3/2
  Gain2/1 -> Scope/1, I1/1
  Fuzzy Logic Controller./1 -> Gain2/1
  Mux/1 -> Fuzzy Logic Controller./1
  vp11/1 -> Sum1/2
  Sum1/1 -> Sum2/2

== matlab function Model_V9/Subsystem3/Subsystem/Amortecedor Magnetorreológico /MR tgh ==
  data: v input; x input; Fb output; i input
function Fb = tgh_model(v,x,i)
c = 1929*i+1232;
k = -1700*i+5100;
alpha = -244*i^2+918*i+32;
beta = 100;
gamma = 0.3*i+0.58;
f0 = -18*i-257;
p = 1.3;
% p = 50;
Fb = p*(k*x+c*v+alpha*tanh(beta*v+gamma*sign(x))+f0);
%Fb = c*v+alpha*tanh(beta*v);

== matlab function Model_V9/Subsystem9/Subsystem/Amortecedor Magnetorreológico /MR tgh ==
  data: v input; x input; Fb output; i input
function Fb = tgh_model(v,x,i)
c = 1929*i+1232;
k = -1700*i+5100;
alpha = -244*i^2+918*i+32;
beta = 100;
gamma = 0.3*i+0.58;
f0 = -18*i-257;
p = 1.3;
% p = 50;
Fb = p*(k*x+c*v+alpha*tanh(beta*v+gamma*sign(x))+f0);
%Fb = c*v+alpha*tanh(beta*v);

== matlab function Model_V9/Subsystem16/Subsystem/Fuzzy Controller/MATLAB Function ==
  data: u input; y output
function y = fcn(u)

if (u > 1)
    y = 1;
else
    y = u;
end

== matlab function Model_V9/Subsystem8/Subsystem/Amortecedor Magnetorreológico /MR tgh ==
  data: v input; x input; Fb output; i input
function Fb = tgh_model(v,x,i)
c = 1929*i+1232;
k = -1700*i+5100;
alpha = -244*i^2+918*i+32;
beta = 100;
gamma = 0.3*i+0.58;
f0 = -18*i-257;
p = 1.3;
% p = 50;
Fb = p*(k*x+c*v+alpha*tanh(beta*v+gamma*sign(x))+f0);
%Fb = c*v+alpha*tanh(beta*v);

== matlab function Model_V9/Subsystem16/Subsystem/Fuzzy Controller/MATLAB Function1 ==
  data: u input; y output
function y = fcn(u)

if (u > 1)
    y = 1;
else
    y = u;
end

== matlab function Model_V9/Subsystem16/Subsystem/Fuzzy Controller/MATLAB Function2 ==
  data: u input; y output
function y = fcn(u)

if (u > 1)
    y = 1;
else
    y = u;
end

== matlab function Model_V9/Subsystem16/Subsystem/Mag Damper /MR tgh ==
  data: v input; x input; Fb output; i input
function Fb = tgh_model(v,x,i)
c = 1929*i+1232;
k = -1700*i+5100;
alpha = -244*i^2+918*i+32;
beta = 100;
gamma = 0.3*i+0.58;
f0 = -18*i-257;
p = 1.3;
% p = 50;
Fb = p*(k*x+c*v+alpha*tanh(beta*v+gamma*sign(x))+f0);
%Fb = c*v+alpha*tanh(beta*v);
